simulink model "PID_fuzzy_sup"  (Simulink 7.1)
settings: Solver=ode3  StartTime=0.0  StopTime=tfinal  FixedStep=0.01  RelTol=1e-3
libraries: fuzblock x3
settings Model: Creator=a2791ft  LastModifiedBy=a2791ft
settings SolverCC: MaxConsecutiveZCs=1e6  ZeroCrossControl=DisableAll

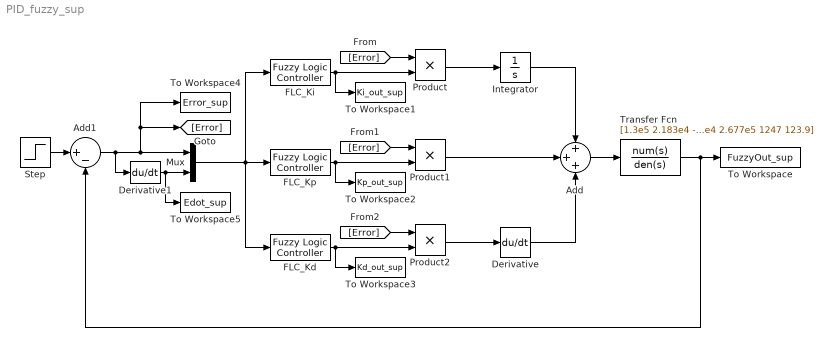
== system PID_fuzzy_sup ==
  Add : Sum  Inputs=+++  OutDataType=sfix(16)  OutScaling=2^-10
  Add1 : Sum  Inputs=|+-  OutDataType=sfix(16)  OutScaling=2^-10
  Derivative : Derivative  LinearizePole=-1
  Derivative1 : Derivative
  FLC_Kd : fuzblock/Fuzzy Logic  Controller  SystemSampleTime=-1  fis=Kdfz
  FLC_Ki : fuzblock/Fuzzy Logic  Controller  SystemSampleTime=-1  fis=Kifz
  FLC_Kp : fuzblock/Fuzzy Logic  Controller  SystemSampleTime=-1  fis=Kpfz
  Integrator : Integrator
  Mux : Mux  Inputs=2
  Product : Product  OutDataType=sfix(16)  OutScaling=2^0  RndMeth=Zero
  Product1 : Product  OutDataType=sfix(16)  OutScaling=2^0  RndMeth=Zero
  Product2 : Product  OutDataType=sfix(16)  OutScaling=2^0  RndMeth=Zero
  Step : Step  SampleTime=0
  To Workspace : ToWorkspace  VariableName=FuzzyOut_sup  SampleTime=-1  SaveFormat=Structure With Time
  To Workspace1 : ToWorkspace  VariableName=Ki_out_sup  SampleTime=-1  SaveFormat=Structure With Time
  To Workspace2 : ToWorkspace  VariableName=Kp_out_sup  SampleTime=-1  SaveFormat=Structure With Time
  To Workspace3 : ToWorkspace  VariableName=Kd_out_sup  SampleTime=-1  SaveFormat=Structure With Time
  To Workspace4 : ToWorkspace  VariableName=Error_sup  SampleTime=-1  SaveFormat=Structure With Time
  To Workspace5 : ToWorkspace  VariableName=Edot_sup  SampleTime=-1  SaveFormat=Structure With Time
  Transfer Fcn : TransferFcn  Numerator=[1.3e5 2.183e4 -31.29]  Denominator=[1742 1.83e4 3.553e4 2.677e5 1247 123.9]
  wires:
  Step/1 -> Add1/1
  Transfer Fcn/1 -> To Workspace/1, Add1/2
  Add/1 -> Transfer Fcn/1
  Mux/1 -> FLC_Kp/1, FLC_Ki/1, FLC_Kd/1
  Integrator/1 -> Add/1
  Derivative/1 -> Add/3
  Add1/1 -> Derivative1/1, Mux/1, [Error], To Workspace4/1
  Derivative1/1 -> Mux/2, To Workspace5/1
  Product/1 -> Integrator/1
  FLC_Ki/1 -> Product/2, To Workspace1/1
  Product1/1 -> Add/2
  FLC_Kp/1 -> Product1/2, To Workspace2/1
  Product2/1 -> Derivative/1
  FLC_Kd/1 -> Product2/2, To Workspace3/1
  [Error] -> Product/1
  [Error] -> Product1/1
  [Error] -> Product2/1
